simulink model "sim_4_newnew"  (R2015b)
settings: Solver=ode45  StartTime=0  StopTime=700  FixedStep=1e-3  RelTol=1e-4
undefined symbols (not defined in the file or in its folder): A, alpha_nc, alpha_nw, B, currentCoeffMatrix, D, E, f, H, h, K2, K3, K4, Kd_surge, Kd_sway, Kd_yaw, Ki_surge, Ki_sway, Ki_yaw, Kp_surge, Kp_sway, Kp_yaw, M_inverse, mu, N_freq, P0, Par, phi, Q, R, S, Sim, T, T_pinv, TA_sampling_time, thrusterPositionX, thrusterPositionY, thrusters, thrustersInitialAlpha, U_mean_c, U_mean_w, windCoeffMatrix, x0
libraries: simulink_extras x15, simulink x10, marine_gnc x5
(part 2 of 2)

== system sim_4_newnew/Vessel Dynamics1/Vessel LF 6DOF/J(Eta)/Tnb_gnc ==
  note: gnc Simulink toolbox
  theta : Inport
  Constant : Constant
  "Constant " : Constant  Value=0
  Mux2 : Mux  Inputs=9
  Reshape 9x1->3x3 : Reshape  OutputDimensionality=Customize  OutputDimensions=[3,3]
  "T21 " : Fcn  Expr=sin(u(1))*tan(u(2))
  T22 : Fcn  Expr=cos(u(1))
  T23 : Fcn  Expr=sin(u(1))/cos(u(2))
  "T31 " : Fcn  Expr=cos(u(1))*tan(u(2))
  T32 : Fcn  Expr=-sin(u(1))
  T33 : Fcn  Expr=cos(u(1))/cos(u(2))
  T : Outport  InitialOutput=0
  wires:
  Constant/1 -> Mux2/1
  Mux2/1 -> Reshape 9x1->3x3/1
  Reshape 9x1->3x3/1 -> T/1
  theta/1 -> "T21 "/1, T22/1, "T31 "/1, T32/1, T33/1, T23/1
  T23/1 -> Mux2/6
  T22/1 -> Mux2/5
  T33/1 -> Mux2/9
  "Constant "/1 -> Mux2/2, Mux2/3
  "T21 "/1 -> Mux2/4
  "T31 "/1 -> Mux2/7
  T32/1 -> Mux2/8

== system sim_4_newnew/Vessel Dynamics1/Vessel LF 6DOF/Rotate_yaw_T/GNC: "Transposed rotation matrix yaw" ==
  note: GNC: "Transposed
      | rotation matrix yaw"
  psi : Inport
  nu : Inport  Port=2  PortDimensions=3
  Fcn : Fcn  Expr=cos(u(1))*u(2)+sin(u(1))*u(3)
  Fcn1 : Fcn  Expr=-sin(u(1))*u(2)+cos(u(1))*u(3)
  Fcn2 : Fcn  Expr=u(4)
  Mux2 : Mux  Inputs=2
  Mux3 : Mux  Inputs=3
  R*nu : Outport
  wires:
  Mux2/1 -> Fcn1/1, Fcn/1, Fcn2/1
  Fcn/1 -> Mux3/1  "x_dot"
  Fcn1/1 -> Mux3/2  "y_dot"
  Fcn2/1 -> Mux3/3  "psi_dot"
  Mux3/1 -> R*nu/1  "eta_dot"
  psi/1 -> Mux2/1
  nu/1 -> Mux2/2

== system sim_4_newnew/Vessel Dynamics1/Vessel LF 6DOF/C_a/C_a calculation/Smtrx_T ==
  note: Transposed S-matrix
  r : Inport
  Mux : Mux  Inputs=9
  Reshape 9x1 => 3x1 : Reshape  OutputDimensionality=Customize  OutputDimensions=[3,3]
  h11 : Fcn  Expr=0
  h12 : Fcn  Expr=u(3)
  h13 : Fcn  Expr=-u(2)
  h21 : Fcn  Expr=-u(3)
  h22 : Fcn  Expr=0
  h23 : Fcn  Expr=u(1)
  h31 : Fcn  Expr=u(2)
  h32 : Fcn  Expr=-u(1)
  h33 : Fcn  Expr=0
  S_T(r) : Outport
  wires:
  r/1 -> h33/1, h23/1, h13/1, h32/1, h22/1, h12/1, h21/1, h11/1, h31/1
  h33/1 -> Mux/9
  h23/1 -> Mux/8
  h13/1 -> Mux/7
  h32/1 -> Mux/6
  h22/1 -> Mux/5
  h12/1 -> Mux/4
  h31/1 -> Mux/3
  h21/1 -> Mux/2
  h11/1 -> Mux/1
  Mux/1 -> Reshape 9x1 => 3x1/1
  Reshape 9x1 => 3x1/1 -> S_T(r)/1

== system sim_4_newnew/Vessel Dynamics1/Vessel LF 6DOF/C_a/C_a calculation/Smtrx_T1 ==
  note: Transposed S-matrix
  r : Inport
  Mux : Mux  Inputs=9
  Reshape 9x1 => 3x1 : Reshape  OutputDimensionality=Customize  OutputDimensions=[3,3]
  h11 : Fcn  Expr=0
  h12 : Fcn  Expr=u(3)
  h13 : Fcn  Expr=-u(2)
  h21 : Fcn  Expr=-u(3)
  h22 : Fcn  Expr=0
  h23 : Fcn  Expr=u(1)
  h31 : Fcn  Expr=u(2)
  h32 : Fcn  Expr=-u(1)
  h33 : Fcn  Expr=0
  S_T(r) : Outport
  wires:
  Reshape 9x1 => 3x1/1 -> S_T(r)/1
  Mux/1 -> Reshape 9x1 => 3x1/1
  h11/1 -> Mux/1
  h21/1 -> Mux/2
  h31/1 -> Mux/3
  h12/1 -> Mux/4
  h22/1 -> Mux/5
  h32/1 -> Mux/6
  h13/1 -> Mux/7
  h23/1 -> Mux/8
  h33/1 -> Mux/9
  r/1 -> h31/1, h11/1, h21/1, h12/1, h22/1, h32/1, h13/1, h23/1, h33/1

== system sim_4_newnew/Vessel Dynamics1/Vessel LF 6DOF/C_rb/C_rb Calculation/Smtrx_T ==
  note: Transposed S-matrix
  r : Inport
  Mux : Mux  Inputs=9
  Reshape 9x1 => 3x1 : Reshape  OutputDimensionality=Customize  OutputDimensions=[3,3]
  h11 : Fcn  Expr=0
  h12 : Fcn  Expr=u(3)
  h13 : Fcn  Expr=-u(2)
  h21 : Fcn  Expr=-u(3)
  h22 : Fcn  Expr=0
  h23 : Fcn  Expr=u(1)
  h31 : Fcn  Expr=u(2)
  h32 : Fcn  Expr=-u(1)
  h33 : Fcn  Expr=0
  S_T(r) : Outport
  wires:
  r/1 -> h22/1, h12/1, h21/1, h11/1, h31/1, h33/1, h23/1, h13/1, h32/1
  h33/1 -> Mux/9
  h23/1 -> Mux/8
  h13/1 -> Mux/7
  h32/1 -> Mux/6
  h22/1 -> Mux/5
  h12/1 -> Mux/4
  h31/1 -> Mux/3
  h21/1 -> Mux/2
  h11/1 -> Mux/1
  Mux/1 -> Reshape 9x1 => 3x1/1
  Reshape 9x1 => 3x1/1 -> S_T(r)/1

== system sim_4_newnew/Vessel Dynamics1/Vessel LF 6DOF/C_rb/C_rb Calculation/Smtrx_T1 ==
  note: Transposed S-matrix
  r : Inport
  Mux : Mux  Inputs=9
  Reshape 9x1 => 3x1 : Reshape  OutputDimensionality=Customize  OutputDimensions=[3,3]
  h11 : Fcn  Expr=0
  h12 : Fcn  Expr=u(3)
  h13 : Fcn  Expr=-u(2)
  h21 : Fcn  Expr=-u(3)
  h22 : Fcn  Expr=0
  h23 : Fcn  Expr=u(1)
  h31 : Fcn  Expr=u(2)
  h32 : Fcn  Expr=-u(1)
  h33 : Fcn  Expr=0
  S_T(r) : Outport
  wires:
  Reshape 9x1 => 3x1/1 -> S_T(r)/1
  Mux/1 -> Reshape 9x1 => 3x1/1
  h11/1 -> Mux/1
  h21/1 -> Mux/2
  h31/1 -> Mux/3
  h12/1 -> Mux/4
  h22/1 -> Mux/5
  h32/1 -> Mux/6
  h13/1 -> Mux/7
  h23/1 -> Mux/8
  h33/1 -> Mux/9
  r/1 -> h31/1, h11/1, h21/1, h12/1, h22/1, h32/1, h13/1, h23/1, h33/1

== matlab function sim_4_newnew/Env_NEW/Current/MATLAB Function ==
  data: alpha2 output; alpha1 input; east input
function alpha2 = fcn(alpha1,east)
if east < 0
    alpha2 = alpha1 + 180;
else
    alpha2 = alpha1;
end

end

== matlab function sim_4_newnew/Env_force1/get current coeffcients ==
  data: alpha input; C output
function C   = CurrentCoefficients( alpha )
persistent C_current
% Initialization of the return parameter
C=zeros(6,1);

if isempty(C_current) % TODO
    
    C_current = [11786 0 0 0 33000.8 0;
                13751 24354 0 -68191.2 38502.8 -571850;
                15322 46496 0 -130188.8 42901.6 -947490;
                16304 70808 0 -198262.4 45651.2 -1270900;
                16304 95206 0 -266576.8 45651.2 -1501300;
                14339 121710 0 -340788 40149.2 -1447700;
                11000 146070 0 -408996 30800 -1179900;
                7268.3 164050 0 -459340 20351.24 -858400;
                3143 174920 0 -489776 8800.4 -500840;
                -1374.8 179300 0 -502040 -3849.44 -107140;
                -5107.6 174850 0 -489580 -14301.28 214290;
                -8839.1 166060 0 -464968 -24749.48 518280;
                -11982 150570 0 -421596 -33549.6 607860;
                -14339 126300 0 -353640 -40149.2 947490;
                -14537 97417 0 -272767.6 -40703.6 947490;
                -12376 68636 0 -192180.8 -34652.8 750880;
                -10410 42066 0 -117784.8 -29148 518470;
                -9427.9 19898 0 -55714.4 -26398.12 249180;
                -9231.9 0 0 0 -25849.32 0;
                -9427.9 -19898 0 55714.4 -26398.12 -249180
                -10410 -42066 0 117784.8 -29148 -518470;
                -12376 -68636 0 192180.8 -34652.8 -750880;
                -14537 -97417 0 272767.6 -40703.6 -947490;
                -14339 -126300 0 353640 -40149.2 -947490;
                -11982 -150570 0 421596 -33549.6 -607860;
                -8839.1 -166060 0 464968 -24749.48 -518280;
                -5107.6 -174850 0 489580 -14301.28 -214290;
                -1374.8 -179300 0 502040 -3849.44 107140;
                3143 -174920 0 489776 8800.4 500840;
                7268.3 -164050 0 459340 20351.24 858400;
                11000 -146070 0 408996 30800 1179900;
                14339 -121710 0 340788 40149.2 1447700;
                16304 -95206 0 266576.8 45651.2 1501300;
                16304 -70808 0 198262.4 45651.2 1270900;
                15322 -46496 0 130188.8 42901.6 947490;
                13751 -24354 0 68191.2 38502.8 571850;
                11786 0 0 0 33000.8 0;];
end








while alpha > 360
    alpha = alpha - 360;
end

while alpha < 0
    alpha = alpha + 360;
end

alpha_mod = mod(alpha,10);
avrundet_alpha = alpha - alpha_mod;
index = avrundet_alpha/10+1;

C1 = C_current(index,:)';
C2 = C_current(index+1,:)';

for i = 1:6
    diff = C2(i)-C1(i);
    point = (diff/10)*alpha_mod;
    C(i) = C1(i)+point;
end

end

== matlab function sim_4_newnew/Env_force1/Wind/length ==
  data: v input; V output
function V = fcn(v)
%#codegen

V = sqrt(v(1)^2 + v(2)^2);
end

== matlab function sim_4_newnew/Env_force1/get wind coeffcients ==
  data: alpha input; C output
function C   = WindCoeffcients( alpha )
persistent C_wind
% Initialization of the return parameter
C=zeros(6,1);

if isempty(C_wind) % TODO
    
    C_wind =    [248.37 0 0 0 -2355.232759 0;
                265.19 61.332 0 275.994 -2514.732759 551.1;
                224.13 136.22 0 612.99 -2125.37069 661.56;
                149.03 238.76 0 1074.42 -1413.215517 451.37;
                134.36 319.42 0 1437.39 -1274.103448 212.51;
                96.8 380.5 0 1712.25 -917.9310345 -23.578;
                41.364 396.1 0 1782.45 -392.2448276 1168.3;
                16.477 372.96 0 1678.32 -156.2474138 2376.3;
                0.30412 376.5 0 1694.25 -2.883896552 3511.9;
                -3.723 390.01 0 1755.045 35.30431034 4610.4;
                -24.879 386.63 0 1739.835 235.9215517 4769.5;
                -61.281 393.76 0 1771.92 581.112931 5921.9;
                -108.5 408.66 0 1838.97 1028.87931 6542.8;
                -169.35 393.26 0 1769.67 1605.905172 6805.2;    
                -206.63 276.93 0 1246.185 1959.422414 6751.5;
                -201.99 200.64 0 902.88 1915.422414 6190.1;
                -196.51 124.71 0 561.195 1863.456897 3758.8;
                -181.53 56.27 0 253.215 1721.405172 1905.6;
                -208.22 0 0 0 1974.5 0;
                -181.53 -56.27 0 -253.215 1721.405172 -1905.6;
                -196.51 -124.71 0 -561.195 1863.456897 -3758.8;
                -201.99 -200.64 0 -902.88 1915.422414 -6190.1;
                -206.63 -276.93 0 -1246.185 1959.422414 -6751.5;
                -169.35 -393.26 0 -1769.67 1605.905172 -6805.2;
                -108.5 -408.66 0 -1838.97 1028.87931 -6542.8;
                -61.281 -393.76 0 -1771.92 581.112931 -5921.9;
                -24.879 -386.63 0 -1739.835 235.9215517 -4769.5;
                -3.723 -390.01 0 -1755.045 35.30431034 -4610.4;
                0.30412 -376.5 0 -1694.25 -2.883896552 -3511.9;
                16.477 -372.96 0 -1678.32 -156.2474138 -2376.3;
                41.364 -396.1 0 -1782.45 -392.2448276 -1168.3;
                96.8 -380.5 0 -1712.25 -917.9310345 23.578;
                134.36 -319.42 0 -1437.39 -1274.103448 -212.51;
                149.03 -238.76 0 -1074.42 -1413.215517 -451.37;
                224.13 -136.22 0 -612.99 -2125.37069 -661.56;
                265.19 -61.332 0 -275.994 -2514.732759 -551.1;
                248.37 0 0 0 -2355.232759 0;];
end






while alpha > 360
    alpha = alpha - 360;
end

while alpha < 0
    alpha = alpha + 360;
end

alpha_mod = mod(alpha,10);
avrundet_alpha = alpha - alpha_mod;
index = avrundet_alpha/10+1;

C1 = C_wind(index,:)';
C2 = C_wind(index+1,:)';

for i = 1:6
    diff = C2(i)-C1(i);
    point = (diff/10)*alpha_mod;
    C(i) = C1(i)+point;
end

end

== matlab function sim_4_newnew/Env_force1/Current/length ==
  data: v input; V output
function V = fcn(v)
%#codegen

V = sqrt(v(1)^2 + v(2)^2);
end

== matlab function sim_4_newnew/Env_force1/Wind/MATLAB Function ==
  data: alpha2 output; alpha1 input; north input
function alpha2 = fcn(alpha1,north)
if north < 0
    alpha2 = alpha1 + pi;
else
    alpha2 = alpha1;
end

end

== matlab function sim_4_newnew/Env_force1/Current/MATLAB Function ==
  data: alpha2 output; alpha1 input; east input
function alpha2 = fcn(alpha1,east)
if east < 0
    alpha2 = alpha1 + 180;
else
    alpha2 = alpha1;
end

end

== matlab function sim_4_newnew/Observer 1/Extended Kalman Filter/Extended Kalman Filter ==
  data: y input; estimatedEtaAndNu output; tau input; Q input; R input; x0 input; P0 input; A input; M_inverse input; B input; E input; H input; h input
function estimatedEtaAndNu = ExtendedKalmanFilter(y,tau, Q, R, x0, P0, A, M_inverse,B, E, H, h)
persistent x_bar
persistent P_bar

if isempty(x_bar) % TODO
    x_bar= x0;
end

if isempty(P_bar) 
    P_bar = P0;
end

%%%%%%%%%%%%%%%%%%%%% Update A matrix%%%%%%%%%%%%%%%%%%%%%%%%%%%%%%%%%
s_psi = sin(x_bar(3));
c_psi = cos(x_bar(3));

R_psi = [   c_psi   -s_psi  0;
            s_psi   c_psi   0;
            0       0       1; ];

A(1:3,7:9) = R_psi;
A(7:9,4:6) = M_inverse*R_psi;
%%%%%%%%%%%%%%%%%%%%%%%%%%%%%%%%%%%%%%%%%%%%%%%%%%%%%%%%%%%%%%%%%%%%%%


%%%%%%%%%%%%%%%%%%%%% Kalman state matrices%%%%%%%%%%%%%%%%%%%%%%%%%%%
PHI=eye(9)+A.*h;
DELTA=(eye(9).*h+0.5.*A.*h.*h)*B;
GAMMA=(eye(9).*h+0.5.*A.*h.*h)*E;
%%%%%%%%%%%%%%%%%%%%%%%%%%%%%%%%%%%%%%%%%%%%%%%%%%%%%%%%%%%%%%%%%%%%%%

%%%%%%%%%%%%%%%%% Kalman algorithm%%%%%%%%%%%%%%%%%%%%%%%%%%%%%%%%%%%%
% Kalman gain matrix
K = P_bar*H'*inv(H*P_bar*H'+R);
% Update state estimate
x_hat = x_bar + K*(y-H*x_bar);
% corrector - compute error covariance
P_hat = (eye(9)-K*H)*P_bar*(eye(9)-K*H)'+K*R*K';

x_bar=PHI*x_hat+DELTA*tau;
P_bar=PHI*P_hat*PHI' + GAMMA*Q*GAMMA';
%%%%%%%%%%%%%%%%%%%%%%%%%%%%%%%%%%%%%%%%%%%%%%%%%%%%%%%%%%%%%%%%%%%%%%

%%%%%%%%%%%%%Output of the desired estimates (eta and nu)%%%%%%%%%%%%%
estimatedEtaAndNu=[x_hat(1);x_hat(2);x_hat(3);x_hat(7);x_hat(8);x_hat(9)];
%%%%%%%%%%%%%%%%%%%%%%%%%%%%%%%%%%%%%%%%%%%%%%%%%%%%%%%%%%%%%%%%%%%%%%
end

== matlab function sim_4_newnew/Env_NEW/Current/length ==
  data: v input; V output
function V = fcn(v)
%#codegen

V = sqrt(v(1)^2 + v(2)^2);
end

== matlab function sim_4_newnew/Env_NEW/Wind/Slowly-varying wind + gust/by using Harris Spectrum ==
  data: S input; Ug output; f input; phi input; N_freq input; t input
function Ug = fcn(S, f, phi, N_freq, t)
Ug = 0; % dummy value due to Ug first defined in for-loop
for i = 1:N_freq
    Ug = Ug + sqrt(2*S(i)*(f(2)-f(1))) * cos(2*pi*f(i)*t + phi(i));
end
end

== matlab function sim_4_newnew/Env_NEW/Wind/get the angle in the 1st and 2nd quadrant ==
  data: alpha2 output; alpha1 input; north input
function alpha2 = fcn(alpha1,north)
if north < 0
    alpha2 = alpha1 + pi;
else
    alpha2 = alpha1;
end

end

== matlab function sim_4_newnew/Env_NEW/get current coeffcients ==
  data: alpha input; C output; currentCoeffMatrix input
function C   = CurrentCoefficients( alpha, currentCoeffMatrix )
% Initialization of the return parameter
C=zeros(6,1);

while alpha > 360
    alpha = alpha - 360;
end

while alpha < 0
    alpha = alpha + 360;
end

alpha_mod = mod(alpha,10);
avrundet_alpha = alpha - alpha_mod;
index = avrundet_alpha/10+1;

C1 = currentCoeffMatrix(index,:)';
C2 = currentCoeffMatrix(index+1,:)';

for i = 1:6
    diff = C2(i)-C1(i);
    point = (diff/10)*alpha_mod;
    C(i) = C1(i)+point;
end

end

== matlab function sim_4_newnew/Env_NEW/get wind coeffcients ==
  data: alpha input; C output; windCoeffMatrix input
function C   = WindCoeffcients(alpha, windCoeffMatrix)
% Initialization of the return parameter
C=zeros(6,1);

while alpha > 360
    alpha = alpha - 360;
end

while alpha < 0
    alpha = alpha + 360;
end

alpha_mod = mod(alpha,10);
avrundet_alpha = alpha - alpha_mod;
index = avrundet_alpha/10+1;

C1 = windCoeffMatrix(index,:)';
C2 = windCoeffMatrix(index+1,:)';

for i = 1:6
    diff = C2(i)-C1(i);
    point = (diff/10)*alpha_mod;
    C(i) = C1(i)+point;
end

end
